simulink model "GDGC5"  (R2025a)
settings: Solver=VariableStepAuto  StartTime=0.0  StopTime=10.0  RelTol=1e-3
libraries: aerolibfltsims x2, instrumentseriallib x2
settings Model: PacingRate=11  Creator=pjpra  LastModifiedBy=pjpra

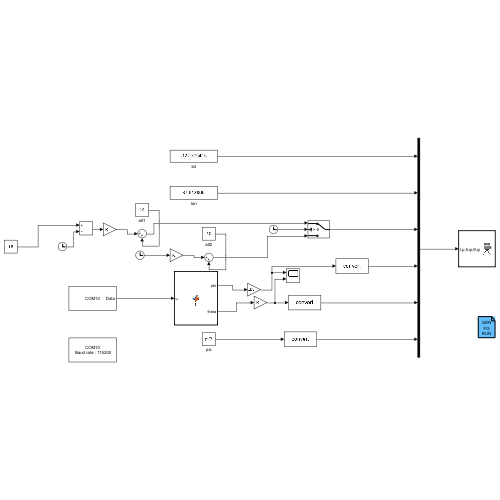
[thumbnail: Simulink's stored preview of the top-level diagram]
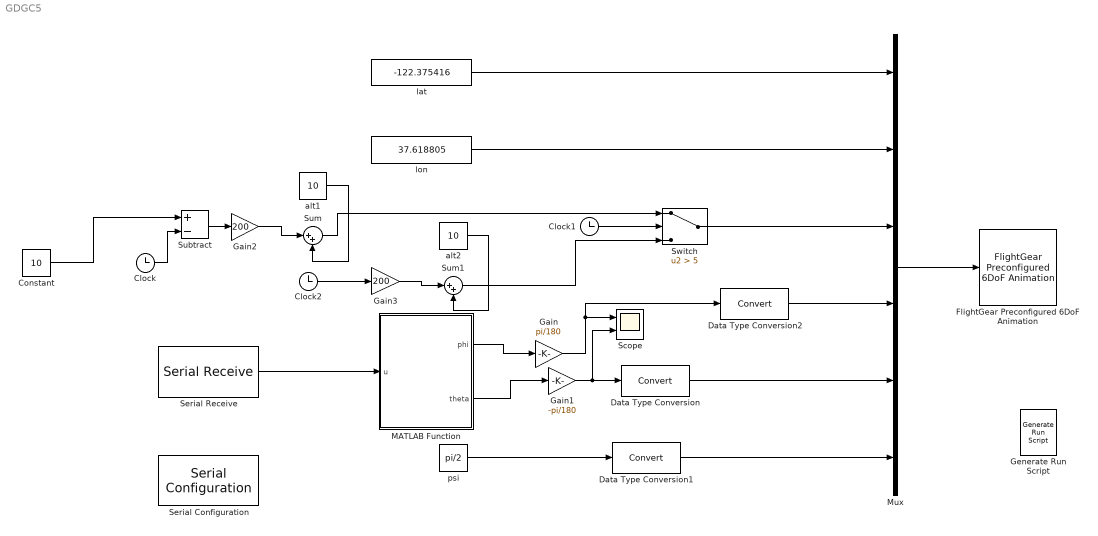
== system GDGC5 ==
  Clock : Clock
  Clock1 : Clock
  Clock2 : Clock
  Constant : Constant  Value=10
  Data Type Conversion : DataTypeConversion  SaturateOnIntegerOverflow=off  RndMeth=Floor
  Data Type Conversion1 : DataTypeConversion  SaturateOnIntegerOverflow=off  RndMeth=Floor
  Data Type Conversion2 : DataTypeConversion  SaturateOnIntegerOverflow=off  RndMeth=Floor
  FlightGear Preconfigured 6DoF Animation : aerolibfltsims/FlightGear Preconfigured 6DoF Animation  xFlightGearVersion=v2019.1  DestinationIpAddress=127.0.0.1  DestinationPort=5502  SampleTime=1/30  packetVersion=24
  Gain : Gain  Gain=pi/180
  Gain1 : Gain  Gain=-pi/180
  Gain2 : Gain  Gain=200
  Gain3 : Gain  Gain=200
  Generate Run Script : aerolibfltsims/Generate Run Script  Architecture=Win64  dataFlow=Send  GeometryModelName=HL21  AirportId=KSFO  RunwayId=10L  InitialAltitude=7224  InitialHeading=113  OffsetDistance=4.72  OffsetAzimuth=0  InstallScenery=off  DisableShaders=off  OriginAddress=127.0.0.1  DestinationPort=5502  OriginPort=5505  LocalAddress=127.0.0.1  OutputFileName=GDGCPPJ1.bat  FlightGearBaseDirectory=C:\Program Files\FlightGear 2019.1.1
  MATLAB Function : MATLAB Function  TreatAsAtomicUnit=on
  Mux : Mux  Inputs=6
  Scope : Scope  NumInputPorts=2
      settings: ActiveDisplayYMinimum=-0.013525344274965552  ActiveDisplayYMaximum=0.023010321200091943
  Serial Configuration : instrumentseriallib/Serial Configuration  Priority=-200000  PortSel=COM10  Port=COM10  ComPort=COM10  BaudRate=115200  DataBits=8  Parity=none  StopBits=1  ByteOrder=little-endian  FlowControl=none  Timeout=10  SimulateUsing=Interpreted execution  BlockInModel=on  aMode=1
      settings: LibrarySourceBlock=embeddedtargetslib/Host Communication/Serial Configuration
  Serial Receive : instrumentseriallib/Serial Receive  Priority=1  PortSel=COM10  Port=COM10  ComPort=COM10  DataType=uint8  SaveDataType=uint8  ToggleHeader=off  Header=[]  ToggleDataSize=on  DataSize=200  ToggleTerminator=off  Terminator=<none>  CustomTerminator=[]  InputFormat=Column major  EnableBlockingMode=on  ActionDataUnavailable=Output last received value  ActionWhenDataUnavailable=Output last received value  CustomValue=0  SampleTime=0.01  SimulateUsing=Interpreted execution  BlockInModel=on  aMode=1  LibraryInUse=instrumentlib
      settings: LibrarySourceBlock=embeddedtargetslib/Host Communication/Serial Receive
  Subtract : Sum  Inputs=+-
  Sum : Sum  Inputs=|++
  Sum1 : Sum  Inputs=|++
  Switch : Switch  Criteria=u2 > Threshold  Threshold=5  SaturateOnIntegerOverflow=off  InputSameDT=off
  alt1 : Constant  Value=10
  alt2 : Constant  Value=10
  lat : Constant  Value=-122.375416
  lon : Constant  Value=37.618805
  psi : Constant  Value=pi/2
  wires:
  Serial Receive/1 -> MATLAB Function/1(u)
  MATLAB Function/1(phi) -> Gain/1
  MATLAB Function/2(theta) -> Gain1/1
  Gain1/1 -> Scope/2, Data Type Conversion/1
  Gain/1 -> Scope/1, Data Type Conversion2/1
  lat/1 -> Mux/1
  lon/1 -> Mux/2
  psi/1 -> Data Type Conversion1/1
  Data Type Conversion/1 -> Mux/5
  Data Type Conversion1/1 -> Mux/6
  Data Type Conversion2/1 -> Mux/4
  Mux/1 -> FlightGear Preconfigured 6DoF Animation/1
  Clock/1 -> Subtract/2
  Gain2/1 -> Sum/1
  alt1/1 -> Sum/2
  Sum/1 -> Switch/1
  Switch/1 -> Mux/3
  Clock1/1 -> Switch/2
  Sum1/1 -> Switch/3
  alt2/1 -> Sum1/2
  Clock2/1 -> Gain3/1
  Gain3/1 -> Sum1/1
  Constant/1 -> Subtract/1
  Subtract/1 -> Gain2/1

== matlab function GDGC5/MATLAB Function ==
  data: u input; phi output double; theta output double
function [phi, theta] = f(u)

persistent phi_prev theta_prev

if isempty(phi_prev)
    phi_prev = 0;
    theta_prev = 0;
end

str = char(u');

phi = phi_prev;
theta = theta_prev;

startIdx = 0;
endIdx = 0;

for i = 1:length(str)
    if str(i) == '<'
        startIdx = i;
    end
    if str(i) == '>'
        endIdx = i;
    end
end

if startIdx == 0 || endIdx == 0 || endIdx <= startIdx
    return;
end

packet = str(startIdx+1:endIdx-1);

commaIdx = 0;
for i = 1:length(packet)
    if packet(i) == ','
        commaIdx = i;
        break;
    end
end

if commaIdx == 0
    return;
end

phi_val   = str2double(packet(1:commaIdx-1));
theta_val = str2double(packet(commaIdx+1:end));

if ~isnan(phi_val) && ~isnan(theta_val)
    phi = real(phi_val);
    theta = real(theta_val);

    % store last good value
    phi_prev = phi;
    theta_prev = theta;
end
